simulink model "Dynamic_model"  (R2021b)
settings: Solver=VariableStepAuto  StartTime=0.0  StopTime=100  MaxStep=0.001  RelTol=1e-3
values from neighbouring files (symbols this model uses):
  A = (J/D) - (m*b*d/D)    (= -24.9)    [parameter_dynamic.m]
  B = mx*thetadot^2*[cos(theta);-sin(theta);0;0;0]    [DD_EOM.m]    (also in parameter_dynamic.m = 50)
  b = 0.5    [parameter_dynamic.m]
  d = 1    [DD_EOM_SIMULATION.m]    (also in parameter_dynamic.m = 0.5)
  D = 1.8    [DD_EOM_SIMULATION.m]    (also in model_parameters_general.m = [m , 0 , -m*ybc; parameter_dynamic.m = 1; robot_dynamics_sim.m = [m , 0 , -m*ybc)
  J = 0.1    [parameter_dynamic.m]
  m = 20    [model_parameters_general.m]    (also in parameter_dynamic.m = 100; robot_dynamics_sim.m = 10)
settings Model: Creator=A0072685  LastModifiedBy=A0072685

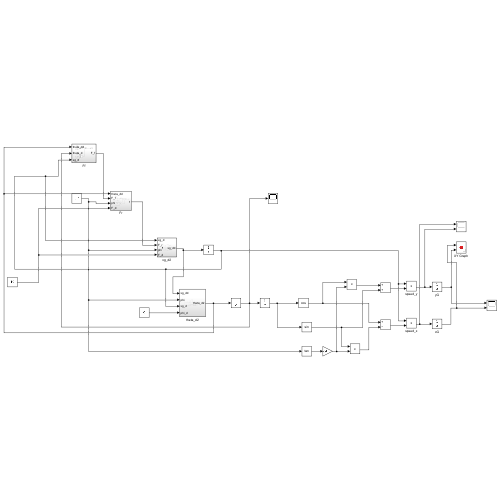
[thumbnail: Simulink's stored preview of the top-level diagram]
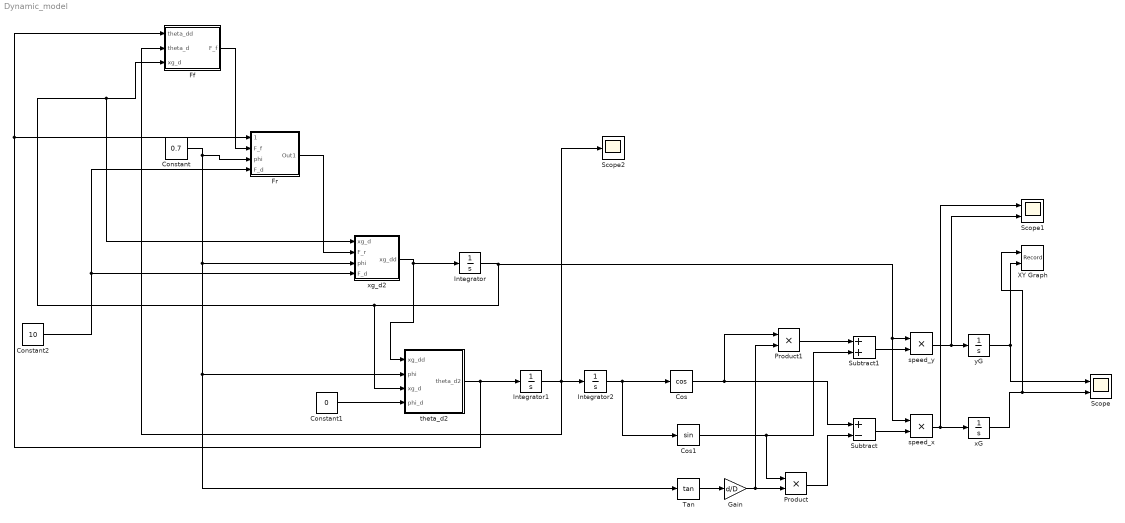
== system Dynamic_model ==
  Constant : Constant  Value=0.7
  Constant1 : Constant  Value=0
  Constant2 : Constant  Value=10
  Cos : Trigonometry  Operator=cos
  Cos1 : Trigonometry
  Ff : Subsystem
  Fr : Subsystem
  Gain : Gain  Gain=d/D
  Integrator : Integrator
  Integrator1 : Integrator
  Integrator2 : Integrator
  Product : Product
  Product1 : Product
  Scope : Scope  NumInputPorts=2
  Scope1 : Scope  NumInputPorts=2
  Scope2 : Scope
  Subtract : Sum  Inputs=+-
  Subtract1 : Sum
  Tan : Trigonometry  Operator=tan
  XY Graph : Record  FileSettingsInternal="{\"entries\":[{\"content\":{\"excelSettings\":{\"content\":{},\"type\":\"Streamout.ExcelSettings\"}},\"type\":\"Streamout.FileSettingStorage\",\"uuid\":\"99e539ef-260c-4b66-b8ba-7e62f2fb5184\"}],\"packageUris\":[\"http://schema.mathworks.com/mf0/streamout_blocks/R2020a\"],\"version\":\"1.0\"}"  Layout=[1 1]  SignalsInternal="{\"entries\":[{\"content\":{\"signals\":[{\"content\":{\"blockPath\":[\"Dynamic_model/XY Graph\"],\"channel\":[],\"dimensions\":[1],\"domain\":\"Dynamic_model/XY Graph\",\"lineColor\":\"#a2142f\",\"plots\":[1],\"port\":1,\"sid\":[\"\"],\"signalID\":5764,\"signalName\":\"xG\"},\"type\":\"RecordBlkView.Signal\",\"uuid\":\"0d65631a-c3c8-4e24-affb-31813795fbf9\"},{\"content\":{\"blockPath\":[\"Dynamic_model/XY Graph\"],\"channel\":[],\"dimensions\":[1],\"domain\":\"Dynamic_model/XY Graph\",\"lineColor\":\"#139fff\",\"plots\":[1],\"port\":2,\"sid\":[\"\"],\"signalID\":5768,\"signalName\":\"yG\"},\"type\":\"RecordBlkView.Signal\",\"uuid\":\"5b886774-f6c1-47d7-80a4-decd86bc44c1\"}]},\"type\":\"RecordBlkView.InputSignals\",\"uuid\":\"b74ae1ec-0f03-4928-ae54-378db1347e74\"}],\"packageUris\":[\"http://schema.mathworks.com/mf0/streamout_blocks/R2020a\"],\"version\":\"1.0\"}"  VisualizationBindings="{\"xyplotplugin\":{\"info\":[{\"series\":[{\"bindingParametersList\":[{\"parameter\":\"X-Axis\",\"signalID\":5764,\"signalName\":\"xG\"},{\"parameter\":\"Y-Axis\",\"signalID\":5768,\"signalName\":\"yG\"}],\"seriesID\":46111}],\"subplotID\":1}]}}"  CompatibilityTag=XY  st=-1
  speed_x : Product
  speed_y : Product
  theta_d2 : Subsystem
  xG : Integrator
  xg_d2 : Subsystem
  yG : Integrator
  wires:
  theta_d2/1(theta_d2) -> Integrator1/1, Ff/1(theta_dd), Fr/1(theta_dd)
  Integrator/1 -> speed_x/1, speed_y/1, theta_d2/3(xg_d), Ff/3(xg_d), xg_d2/1(xg_d)
  Ff/1(F_f) -> Fr/2(F_f)
  Fr/1(Out1) -> xg_d2/2(F_r)
  xg_d2/1(xg_dd) -> theta_d2/1(xg_dd), Integrator/1
  Integrator1/1 -> Scope2/1, Ff/2(theta_d), Integrator2/1
  Integrator2/1 -> Cos1/1, Cos/1
  Tan/1 -> Gain/1
  Gain/1 -> Product1/2, Product/2
  Cos1/1 -> Subtract1/2, Product/1
  Product/1 -> Subtract/2
  Cos/1 -> Product1/1, Subtract/1
  Product1/1 -> Subtract1/1
  Subtract1/1 -> speed_y/2
  Subtract/1 -> speed_x/2
  speed_y/1 -> Scope1/2, yG/1
  speed_x/1 -> Scope1/1, xG/1
  yG/1 -> XY Graph/2, Scope/1
  xG/1 -> XY Graph/1, Scope/2
  Constant2/1 -> xg_d2/4(F_d), Fr/4(F_d)
  Constant/1 -> Tan/1, theta_d2/2(phi), xg_d2/3(phi), Fr/3(phi)
  Constant1/1 -> theta_d2/4(phi_d)

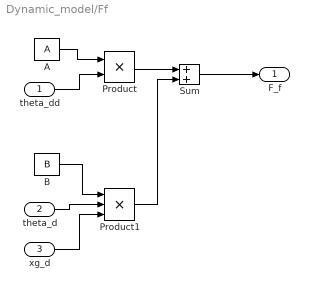
== system Dynamic_model/Ff ==
  theta_dd : Inport
  theta_d : Inport  Port=2
  xg_d : Inport  Port=3
  A : Constant  Value=A
  B : Constant  Value=B
  Product : Product
  Product1 : Product  Inputs=3
  Sum : Sum
  F_f : Outport
  wires:
  theta_dd/1 -> Product/2
  Product1/1 -> Sum/2
  xg_d/1 -> Product1/3
  A/1 -> Product/1
  theta_d/1 -> Product1/2
  B/1 -> Product1/1
  Product/1 -> Sum/1
  Sum/1 -> F_f/1

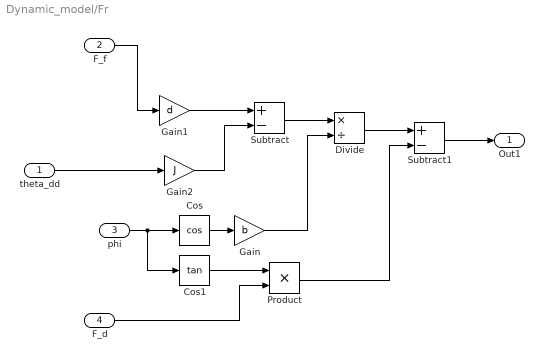
== system Dynamic_model/Fr ==
  theta_dd : Inport
  F_f : Inport  Port=2
  phi : Inport  Port=3
  F_d : Inport  Port=4
  Cos : Trigonometry  Operator=cos
  Cos1 : Trigonometry  Operator=tan
  Divide : Product  Inputs=*/
  Gain : Gain  Gain=b
  Gain1 : Gain  Gain=d
  Gain2 : Gain  Gain=J
  Product : Product
  Subtract : Sum  Inputs=+-
  Subtract1 : Sum  Inputs=+-
  Out1 : Outport
  wires:
  Gain2/1 -> Subtract/2
  Subtract/1 -> Divide/1
  Gain/1 -> Divide/2
  Cos/1 -> Gain/1
  theta_dd/1 -> Gain2/1
  phi/1 -> Cos1/1, Cos/1
  Gain1/1 -> Subtract/1
  Subtract1/1 -> Out1/1
  F_f/1 -> Gain1/1
  Divide/1 -> Subtract1/1
  Cos1/1 -> Product/1
  F_d/1 -> Product/2
  Product/1 -> Subtract1/2

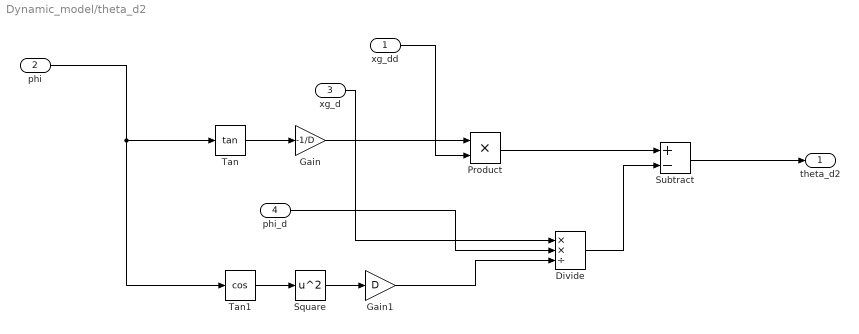
== system Dynamic_model/theta_d2 ==
  xg_dd : Inport
  phi : Inport  Port=2
  xg_d : Inport  Port=3
  phi_d : Inport  Port=4
  Divide : Product  Inputs=**/
  Gain : Gain  Gain=-1/D
  Gain1 : Gain  Gain=D
  Product : Product
  Square : Math  Operator=square  SaturateOnIntegerOverflow=on
  Subtract : Sum  Inputs=+-
  Tan : Trigonometry  Operator=tan
  Tan1 : Trigonometry  Operator=cos
  theta_d2 : Outport
  wires:
  xg_d/1 -> Divide/1
  Square/1 -> Gain1/1
  Subtract/1 -> theta_d2/1
  Gain/1 -> Product/1
  Tan/1 -> Gain/1
  phi/1 -> Tan1/1, Tan/1
  Gain1/1 -> Divide/3
  Product/1 -> Subtract/1
  Tan1/1 -> Square/1
  Divide/1 -> Subtract/2
  xg_dd/1 -> Product/2
  phi_d/1 -> Divide/2

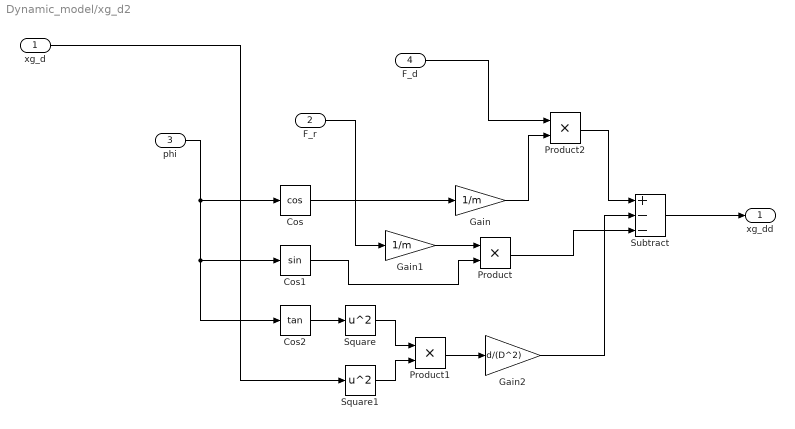
== system Dynamic_model/xg_d2 ==
  xg_d : Inport
  F_r : Inport  Port=2
  phi : Inport  Port=3
  F_d : Inport  Port=4
  Cos : Trigonometry  Operator=cos
  Cos1 : Trigonometry
  Cos2 : Trigonometry  Operator=tan
  Gain : Gain  Gain=1/m
  Gain1 : Gain  Gain=1/m
  Gain2 : Gain  Gain=d/(D^2)
  Product : Product
  Product1 : Product
  Product2 : Product
  Square : Math  Operator=square  SaturateOnIntegerOverflow=on
  Square1 : Math  Operator=square  SaturateOnIntegerOverflow=on
  Subtract : Sum  Inputs=+--
  xg_dd : Outport
  wires:
  Product/1 -> Subtract/3
  Gain2/1 -> Subtract/2
  xg_d/1 -> Square1/1
  Cos2/1 -> Square/1
  Square1/1 -> Product1/2
  Square/1 -> Product1/1
  phi/1 -> Cos2/1, Cos1/1, Cos/1
  Cos1/1 -> Product/2
  Gain1/1 -> Product/1
  F_r/1 -> Gain1/1
  Cos/1 -> Gain/1
  Product1/1 -> Gain2/1
  Subtract/1 -> xg_dd/1
  F_d/1 -> Product2/1
  Gain/1 -> Product2/2
  Product2/1 -> Subtract/1
